simulink model "Coolnt"  (R2018a)
settings: configuration reference "cs_ert" (kept outside this file)
settings Model: DataDictionary=Coolnt.sldd  Creator=zhoutinglin  LastModifiedBy=zhoutinglin

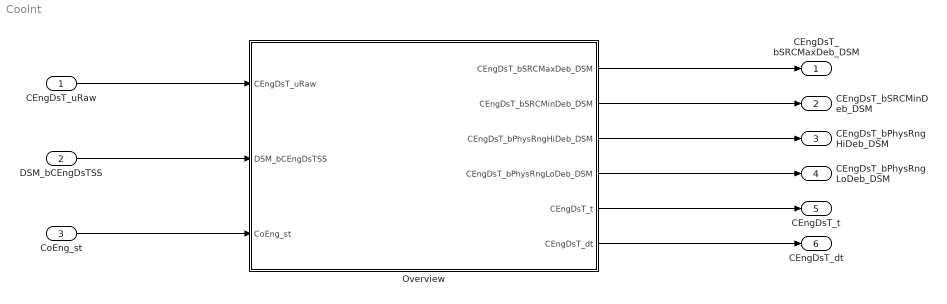
== system Coolnt ==
  CEngDsT_uRaw : Inport
  DSM_bCEngDsTSS : Inport  Port=2
  CoEng_st : Inport  Port=3
  Overview : Subsystem
  CEngDsT_bSRCMaxDeb_DSM : Outport
  CEngDsT_bSRCMinDeb_DSM : Outport  Port=2
  CEngDsT_bPhysRngHiDeb_DSM : Outport  Port=3
  CEngDsT_bPhysRngLoDeb_DSM : Outport  Port=4
  CEngDsT_t : Outport  Port=5
  CEngDsT_dt : Outport  Port=6
  wires:
  CEngDsT_uRaw/1 -> Overview/1(CEngDsT_uRaw)
  DSM_bCEngDsTSS/1 -> Overview/2(DSM_bCEngDsTSS)
  CoEng_st/1 -> Overview/3(CoEng_st)
  Overview/1(CEngDsT_bSRCMaxDeb_DSM) -> CEngDsT_bSRCMaxDeb_DSM/1
  Overview/2(CEngDsT_bSRCMinDeb_DSM) -> CEngDsT_bSRCMinDeb_DSM/1
  Overview/3(CEngDsT_bPhysRngHiDeb_DSM) -> CEngDsT_bPhysRngHiDeb_DSM/1
  Overview/4(CEngDsT_bPhysRngLoDeb_DSM) -> CEngDsT_bPhysRngLoDeb_DSM/1
  Overview/5(CEngDsT_t) -> CEngDsT_t/1
  Overview/6(CEngDsT_dt) -> CEngDsT_dt/1

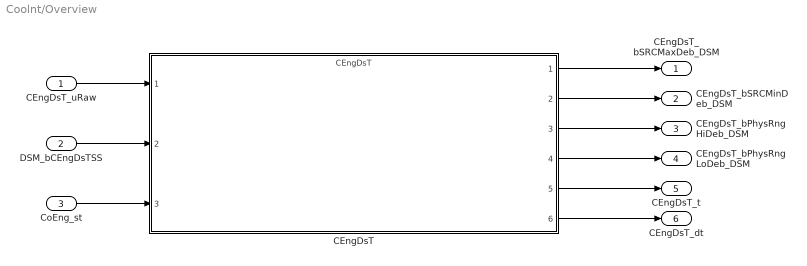
== system Coolnt/Overview ==
  CEngDsT_uRaw : Inport
  DSM_bCEngDsTSS : Inport  Port=2
  CoEng_st : Inport  Port=3
  CEngDsT : ModelReference  ModelNameDialog=CEngDsT  SimulationMode=Normal  ModelReferenceVersion=1.12
  CEngDsT_bSRCMaxDeb_DSM : Outport
  CEngDsT_bSRCMinDeb_DSM : Outport  Port=2
  CEngDsT_bPhysRngHiDeb_DSM : Outport  Port=3
  CEngDsT_bPhysRngLoDeb_DSM : Outport  Port=4
  CEngDsT_t : Outport  Port=5
  CEngDsT_dt : Outport  Port=6
  wires:
  CEngDsT_uRaw/1 -> CEngDsT/1
  DSM_bCEngDsTSS/1 -> CEngDsT/2
  CoEng_st/1 -> CEngDsT/3
  CEngDsT/1 -> CEngDsT_bSRCMaxDeb_DSM/1
  CEngDsT/2 -> CEngDsT_bSRCMinDeb_DSM/1
  CEngDsT/3 -> CEngDsT_bPhysRngHiDeb_DSM/1
  CEngDsT/4 -> CEngDsT_bPhysRngLoDeb_DSM/1
  CEngDsT/5 -> CEngDsT_t/1
  CEngDsT/6 -> CEngDsT_dt/1
